simulink model "handSim"  (R2015b)
settings: Solver=VariableStepAuto  StartTime=0.0  StopTime=1  RelTol=1e-3
settings Model: Creator=Ricardo  LastModifiedBy=Ricardo

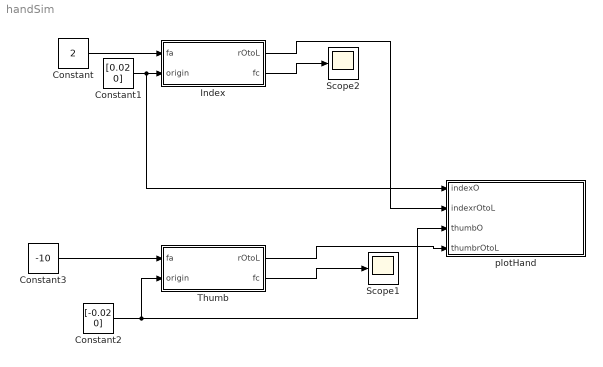
== system handSim ==
  Constant : Constant  Value=2
  Constant1 : Constant  Value=[0.02 0]
  Constant2 : Constant  Value=[-0.02 0]
  Constant3 : Constant  Value=-10
  Index : Subsystem
  Scope1 : Scope
  Scope2 : Scope
  Thumb : Subsystem
  plotHand : MATLAB Function  TreatAsAtomicUnit=on
  wires:
  Constant1/1 -> plotHand/1(indexO), Index/2(origin)
  Constant/1 -> Index/1(fa)
  Index/1(rOtoL) -> plotHand/2(indexrOtoL)
  Index/2(fc) -> Scope2/1
  Constant3/1 -> Thumb/1(fa)
  Constant2/1 -> plotHand/3(thumbO), Thumb/2(origin)
  Thumb/1(rOtoL) -> plotHand/4(thumbrOtoL)
  Thumb/2(fc) -> Scope1/1

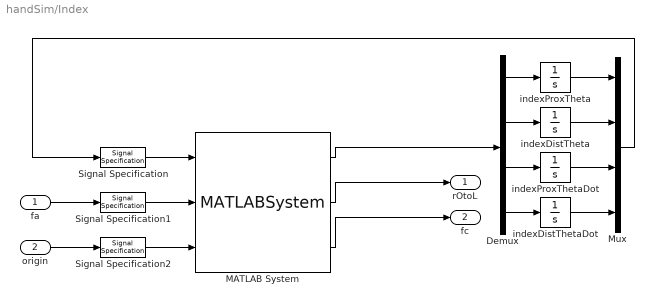
== system handSim/Index ==
  fa : Inport
  origin : Inport  Port=2
  Demux : Demux
  MATLAB System : MATLABSystem  System=Index  kP=-0.043  kD=-0.185  dP=-0.01  dD=-0.01  lP=0.1  lD=0.1  rP=0.02  rD=0.012  mP=0.02  mD=0.02  thetaP=pi/10  thetaD=pi/3  SimulateUsing=Interpreted execution
      mask Type: Index
      mask Display:
      | disp('Index');
      | port_label('input',1,'initVal');
      | port_label('input',2,'fa');
      | port_label('input',3,'origin');
      | port_label('output',1,'xDot');
      | port_label('output',2,'rOtoL');
      | port_label('output',3,'fc');
  Mux : Mux
  Signal Specification : SignalSpecification  Dimensions=4
  Signal Specification1 : SignalSpecification  Dimensions=1
  Signal Specification2 : SignalSpecification  Dimensions=2
  indexDistTheta : Integrator  InitialCondition=pi/3  ContinuousStateAttributes='indexDistTheta'
  indexDistThetaDot : Integrator  ContinuousStateAttributes='indexDistThetaDot'
  indexProxTheta : Integrator  InitialCondition=pi/10  ContinuousStateAttributes='indexProxTheta'
  indexProxThetaDot : Integrator  ContinuousStateAttributes='indexProxThetaDot'
  rOtoL : Outport
  fc : Outport  Port=2
  wires:
  Demux/1 -> indexProxTheta/1
  Demux/2 -> indexDistTheta/1
  Demux/3 -> indexProxThetaDot/1
  Demux/4 -> indexDistThetaDot/1
  MATLAB System/1 -> Demux/1
  indexProxTheta/1 -> Mux/1
  indexDistTheta/1 -> Mux/2
  indexProxThetaDot/1 -> Mux/3
  indexDistThetaDot/1 -> Mux/4
  Mux/1 -> Signal Specification/1
  Signal Specification/1 -> MATLAB System/1
  MATLAB System/2 -> rOtoL/1
  MATLAB System/3 -> fc/1
  Signal Specification1/1 -> MATLAB System/2
  fa/1 -> Signal Specification1/1
  origin/1 -> Signal Specification2/1
  Signal Specification2/1 -> MATLAB System/3

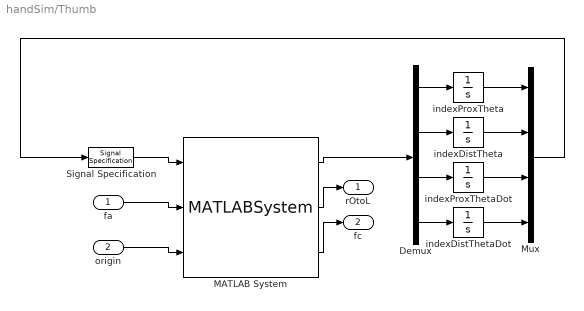
== system handSim/Thumb ==
  fa : Inport
  origin : Inport  Port=2
  Demux : Demux
  MATLAB System : MATLABSystem  System=Thumb  kP=-1  kD=-5  dP=-0.01  dD=-0.01  lP=0.1  lD=0.1  rP=0.02  rD=0.012  mP=0.02  mD=0.02  thetaP=pi-pi/10  thetaD=-pi/3  SimulateUsing=Interpreted execution
      mask Type: Thumb
      mask Display:
      | disp('Thumb');
      | port_label('input',1,'initVal');
      | port_label('input',2,'fa');
      | port_label('input',3,'origin');
      | port_label('output',1,'xDot');
      | port_label('output',2,'rOtoL');
      | port_label('output',3,'fc');
  Mux : Mux
  Signal Specification : SignalSpecification  Dimensions=4
  indexDistTheta : Integrator  InitialCondition=-pi/3  ContinuousStateAttributes='indexDistTheta'
  indexDistThetaDot : Integrator  ContinuousStateAttributes='indexDistThetaDot'
  indexProxTheta : Integrator  InitialCondition=pi-pi/10  ContinuousStateAttributes='indexProxTheta'
  indexProxThetaDot : Integrator  ContinuousStateAttributes='indexProxThetaDot'
  rOtoL : Outport
  fc : Outport  Port=2
  wires:
  Demux/1 -> indexProxTheta/1
  Demux/2 -> indexDistTheta/1
  Demux/3 -> indexProxThetaDot/1
  Demux/4 -> indexDistThetaDot/1
  MATLAB System/1 -> Demux/1
  fa/1 -> MATLAB System/2
  indexProxTheta/1 -> Mux/1
  indexDistTheta/1 -> Mux/2
  indexProxThetaDot/1 -> Mux/3
  indexDistThetaDot/1 -> Mux/4
  Mux/1 -> Signal Specification/1
  Signal Specification/1 -> MATLAB System/1
  MATLAB System/2 -> rOtoL/1
  MATLAB System/3 -> fc/1
  origin/1 -> MATLAB System/3

== matlab function handSim/plotHand ==
  data: indexO input; indexrOtoL input; thumbO input; thumbrOtoL input
% Plots the entire hand to the default figure. Handled in Simulink.
% Author: Ricardo Garcia Rosas
% Change log:
%%%%%%%%%%%%|%%%%%%%%%%%|%%%%%%%%%%%%%%%%%%%%%%%%%%%%%%%%%%%%%%%%%%%|
% Date      |   Author  | Notes                                     |
% 16/03/23  |   RGR     | Added more comments.                      |
function plotHand(indexO,indexrOtoL,thumbO,thumbrOtoL)
    % Plots the entire hand to the default figure. Handled in Simulink.
    % @param indexO Index finger origin position [x,y] (m).
    % @param indexrOtoL Index finger vector from its origin to its link
    % ends.
    % @param thumbO Thumb origin position [x,y] (m).
    % @param thumbrOtoL Thumb vector from its origin to its link ends.

    % Call figure
    figure(1);
    clf;
    hold on;
    % Draw pam
    plot([indexO(1) thumbO(1)],[indexO(2) thumbO(2)],'LineWidth',8,'Color', 'k');
    % Draw Proximal components of Index
    plot([indexO(1) indexrOtoL(1,1)],[indexO(2) indexrOtoL(2,1)],'LineWidth',8,'Color', 'k');
    plot(indexO(1),indexO(2),'ko','MarkerSize',18);
    % Draw Distal components of Index
    plot([indexrOtoL(1,1) indexrOtoL(1,2)],[indexrOtoL(2,1) indexrOtoL(2,2)],'LineWidth',8,'Color', 'k');
    plot(indexrOtoL(1,1),indexrOtoL(2,1),'ko','MarkerSize',18);
    % Draw Index fingertip
    plot(indexrOtoL(1,2),indexrOtoL(2,2),'ko','MarkerSize',8);
    % Draw Proximal components of Thumb
    plot([thumbO(1) thumbrOtoL(1,1)],[thumbO(2) thumbrOtoL(2,1)],'LineWidth',8,'Color', 'k');
    plot(thumbO(1),thumbO(2),'ko','MarkerSize',18);
    % Draw Distal components of Thumn
    plot([thumbrOtoL(1,1) thumbrOtoL(1,2)],[thumbrOtoL(2,1) thumbrOtoL(2,2)],'LineWidth',8,'Color', 'k');
    plot(thumbrOtoL(1,1),thumbrOtoL(2,1),'ko','MarkerSize',18);
    % Draw Thumb fingertip
    plot(thumbrOtoL(1,2),thumbrOtoL(2,2),'ko','MarkerSize',8);
    hold off;
    axis([-0.2 0.2 -0.05 0.2]);
end
